simulink model "COM"  (R2020a)
settings: Solver=FixedStepAuto  StartTime=0.0  StopTime=10.0  FixedStep=1e-3  RelTol=1e-3  EnableMultiTasking=on
undefined symbols (not defined in the file): A0, A1, D13, PTB2, PTB3, PTD1
libraries: frdmk64flib x5, etargetslib x2
settings Model: ExtModeTrigDuration=5  Creator=theodor  LastModifiedBy=theodor
settings OptimizationCC: EnhancedBackFolding=on  PassReuseOutputArgsAs=Individual arguments  ZeroExternalMemoryAtStartup=off  ZeroInternalMemoryAtStartup=off  MaxStackSize=64  OptimizeBlockOrder=speed  DifferentSizesBufferReuse=on  OptimizationCustomize=off  EfficientTunableParamExpr=on
settings DebuggingCC: ParameterTunabilityLossMsg=error
settings HardwareCC: ProdBitPerPointer=32  ProdBitPerSizeT=32  ProdBitPerPtrDiffT=32  ProdLargestAtomicInteger=Long  ProdLargestAtomicFloat=Double  ProdWordSize=32  ProdHWDeviceType=ARM Compatible->ARM Cortex
settings SFSimCC: MATLABDynamicMemAlloc=off
settings RTWCC: SystemTargetFile=ert.tlc  HardwareBoard=NXP FRDM-K64F  TemplateMakefile=ert_default_tmf  Toolchain=GNU Tools for ARM Embedded Processors
settings CodeAppCC: ForceParamTrailComments=on  IgnoreCustomStorageClasses=off  OperatorAnnotations=on  SimulinkDataObjDesc=on  SFDataObjDesc=on  InsertBlockDesc=on

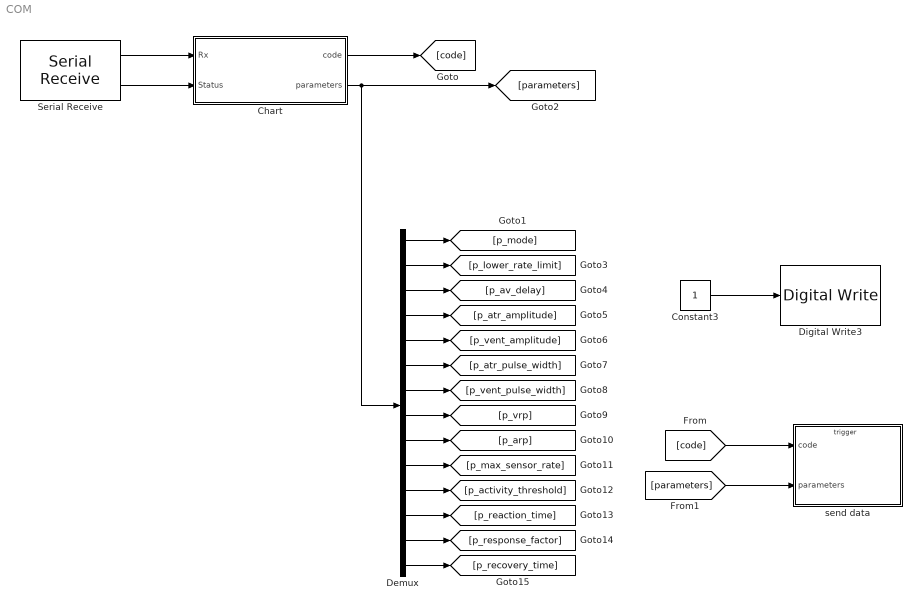
== system COM ==
  Chart : Stateflow chart  TreatAsAtomicUnit=on
  Constant3 : Constant  OutDataTypeStr=uint8
  Demux : Demux  Outputs=14
  Digital Write3 : frdmk64flib/Digital Write  Whichpin=PTD1 (D13)
  Serial Receive : frdmk64flib/Serial Receive  SCIModule=0  Baudrate=uint32(9600)  Parity=None  StopBits=1  HardwareFlowControl=None  ByteOrder=LittleEndian  DataType=uint8  DataLength=15  BlockingMode=off  OutputStatus=on  SampleTime=-1
  send data : Subsystem
  wires:
  Chart/2(parameters) -> Demux/1, [parameters]
  Serial Receive/2 -> Chart/2(Status)
  Serial Receive/1 -> Chart/1(Rx)
  Chart/1(code) -> [code]
  [parameters] -> send data/2(parameters)
  [code] -> send data/1(code)
  Constant3/1 -> Digital Write3/1
  Demux/6 -> [p_atr_pulse_width]
  Demux/5 -> [p_vent_amplitude]
  Demux/4 -> [p_atr_amplitude]
  Demux/3 -> [p_av_delay]
  Demux/2 -> [p_lower_rate_limit]
  Demux/1 -> [p_mode]
  Demux/7 -> [p_vent_pulse_width]
  Demux/8 -> [p_vrp]
  Demux/9 -> [p_arp]
  Demux/10 -> [p_max_sensor_rate]
  Demux/11 -> [p_activity_threshold]
  Demux/12 -> [p_reaction_time]
  Demux/13 -> [p_response_factor]
  Demux/14 -> [p_recovery_time]

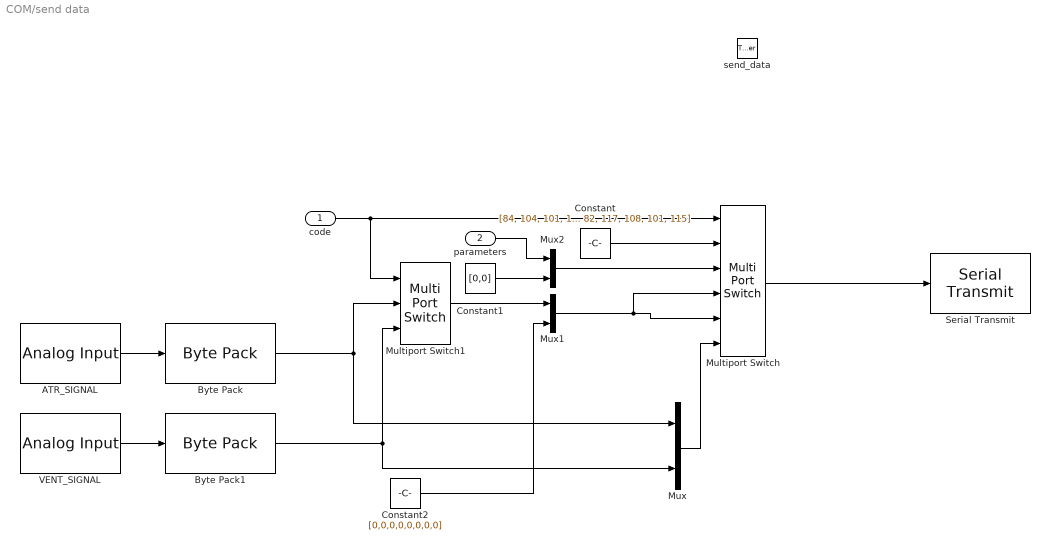
== system COM/send data ==
  code : Inport
  parameters : Inport  Port=2
  send_data : TriggerPort  TriggerType=function-call  IsSimulinkFunction=on  FunctionName=send_data  VariantControl=Variant  PortDimensions=1
  ATR_SIGNAL : frdmk64flib/Analog Input  Whichpin=PTB2 (A0)  SampleTime=-1
  Byte Pack : etargetslib/Byte Pack  datatypes={'double'}  byteAlign=1
  Byte Pack1 : etargetslib/Byte Pack  datatypes={'double'}  byteAlign=1
  Constant : Constant  Value=[84, 104, 101, 111, 100, 111, 114, 65, 111, 107, 105, 82, 117, 108, 101, 115]  OutDataTypeStr=uint8
  Constant1 : Constant  Value=[0,0]
  Constant2 : Constant  Value=[0,0,0,0,0,0,0,0]  OutDataTypeStr=uint8
  Multiport Switch : MultiPortSwitch  DataPortOrder=Specify indices  DataPortIndices={0,2,3,4,5}
  Multiport Switch1 : MultiPortSwitch  DataPortOrder=Specify indices  DataPortIndices={3,4}
  Mux : Mux  Inputs=2
  Mux1 : Mux  Inputs=2
  Mux2 : Mux  Inputs=2
  Serial Transmit : frdmk64flib/Serial Transmit  SCIModule=0  Baudrate=uint32(9600)  Parity=None  StopBits=1  HardwareFlowControl=None  ByteOrder=LittleEndian  BlockingMode=on  OutputStatus=off
  VENT_SIGNAL : frdmk64flib/Analog Input  Whichpin=PTB3 (A1)  SampleTime=-1
  wires:
  ATR_SIGNAL/1 -> Byte Pack/1
  VENT_SIGNAL/1 -> Byte Pack1/1
  code/1 -> Multiport Switch1/1, Multiport Switch/1
  Constant/1 -> Multiport Switch/2
  Byte Pack/1 -> Multiport Switch1/2, Mux/1
  Byte Pack1/1 -> Multiport Switch1/3, Mux/2
  Mux/1 -> Multiport Switch/6
  Multiport Switch/1 -> Serial Transmit/1
  Mux1/1 -> Multiport Switch/5, Multiport Switch/4
  Constant2/1 -> Mux1/2
  Multiport Switch1/1 -> Mux1/1
  Constant1/1 -> Mux2/2
  parameters/1 -> Mux2/1
  Mux2/1 -> Multiport Switch/3

== stateflow chart COM/Chart ==
  state SEND_DATA
    entry:
    code = Rx(1);
    send_data();
  state INITIAL
  state IDLE
  state READ_DATA
    entry:
    code = 1;
    parameters = Rx(2:15);
  (junction 39) -> (junction 41)
  (junction 41) -> IDLE : [Status==32]
  (junction 36) -> (junction 39)
  (default) -> INITIAL
  (junction 27) -> SEND_DATA [order 2]
  SEND_DATA -> (junction 36)
  INITIAL -> IDLE
  IDLE -> (junction 27) : [Status == 0]
  (junction 27) -> READ_DATA [order 1] : [Rx(1)==1]
  READ_DATA -> (junction 36)
  data: code output uint8; Rx input uint8 size=15; Status input uint8; parameters output uint8 size=14
